simulink model "RLS2_1_Stp"  (R2024a)
settings: Solver=FixedStepAuto  StartTime=0.0  StopTime=1000  FixedStep=0.3  RelTol=1e-3
settings Model: Creator=mergenelos  LastModifiedBy=mergenelos

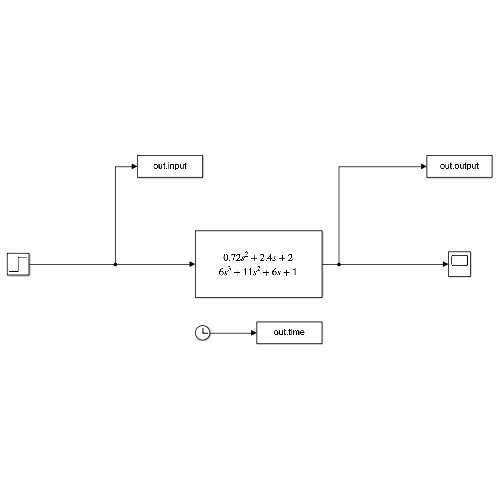
[thumbnail: Simulink's stored preview of the top-level diagram]
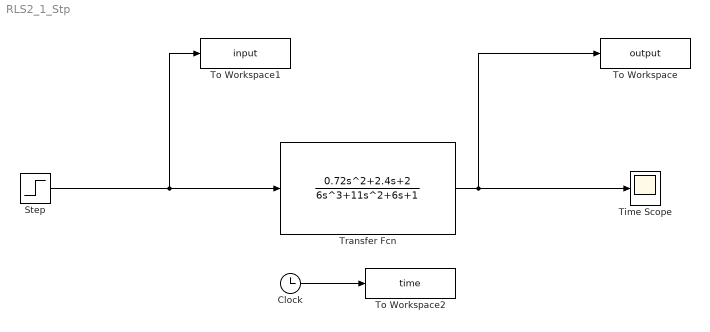
== system RLS2_1_Stp ==
  Clock : Clock
  Step : Step  Time=0  After=2  SampleTime=0
  Time Scope : Scope
  To Workspace : ToWorkspace  VariableName=output  SaveFormat=Timeseries  SampleTime=-1
  To Workspace1 : ToWorkspace  VariableName=input  SaveFormat=Timeseries  SampleTime=-1
  To Workspace2 : ToWorkspace  VariableName=time  SaveFormat=Timeseries  SampleTime=-1
  Transfer Fcn : TransferFcn  Numerator=[0.72 2.4 2]  Denominator=[6 11 6 1]
  wires:
  Transfer Fcn/1 -> To Workspace/1, Time Scope/1
  Clock/1 -> To Workspace2/1
  Step/1 -> To Workspace1/1, Transfer Fcn/1
